simulink model "Punto4"  (R2025b)
settings: Solver=FixedStepAuto  StartTime=0.0  StopTime=60  FixedStep=1e-7  RelTol=1e-3
values from neighbouring files (symbols this model uses):
  A = zeros(2,2)    [Matlab_Traccia_B_(2).m]    (also in PROGETTO_CAT_TRACCIA_B_2.m; Punti_1_2_riscaldatore.m = [A11  A12; Punto_1_riscaldatore.m = [A11  A12; THEULTIMAEONE.m)
  B = zeros(2,1)    [Matlab_Traccia_B_(2).m]    (also in PROGETTO_CAT_TRACCIA_B_2.m; Punti_1_2_riscaldatore.m = [B1; Punto_1_riscaldatore.m = [B1; THEULTIMAEONE.m)
  C = [0 1]    [Matlab_Traccia_B_(2).m]    (also in PROGETTO_CAT_TRACCIA_B_2.m; Punti_1_2_riscaldatore.m; Punto_1_riscaldatore.m; THEULTIMAEONE.m)
  D = 0    [Matlab_Traccia_B_(2).m]    (also in PROGETTO_CAT_TRACCIA_B_2.m; Punti_1_2_riscaldatore.m; Punto_1_riscaldatore.m; THEULTIMAEONE.m)
libraries: cstblocks x1
settings Model: Creator=alex  LastModifiedBy=alex

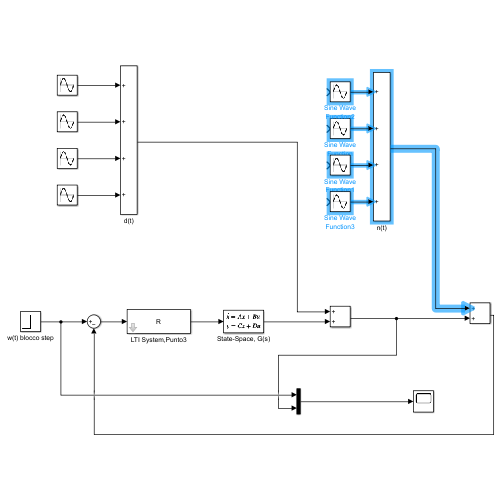
[thumbnail: Simulink's stored preview of the top-level diagram]
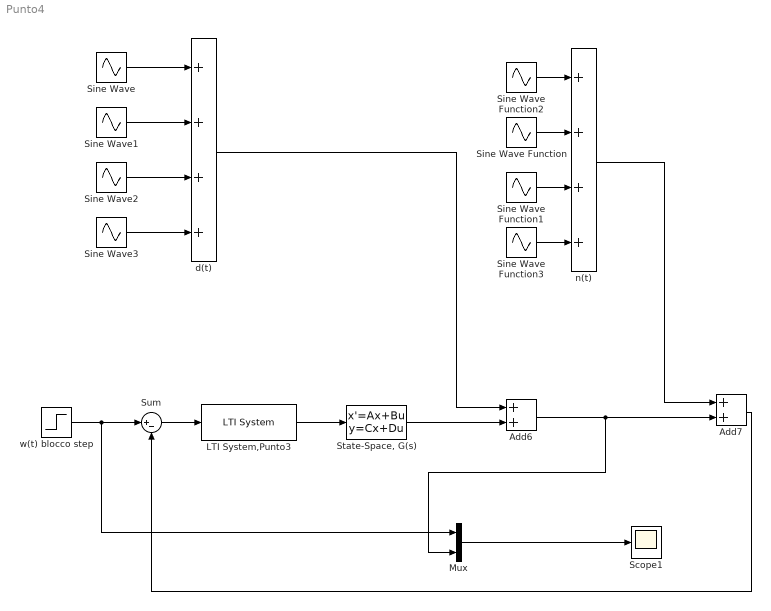
== system Punto4 ==
  Add6 : Sum
  Add7 : Sum
  LTI System,Punto3 : cstblocks/LTI System  sys=R  IC=[]  PadeOrder=0
  Mux : Mux  Inputs=2
  Scope1 : Scope
      settings: ActiveDisplayYMinimum=2.3064084257449133  ActiveDisplayYMaximum=3.4959386286082776  DataLoggingVariableName=sim_out
  Sine Wave : Sin  Amplitude=1.5  Frequency=0.08  SampleTime=0
  Sine Wave Function : Sin  TimeSource=Use external signal  Amplitude=0  Frequency=10e4  SampleTime=0
  Sine Wave Function1 : Sin  TimeSource=Use external signal  Amplitude=0  Frequency=15e4  SampleTime=0
  Sine Wave Function2 : Sin  TimeSource=Use external signal  Amplitude=0  Frequency=5e4  SampleTime=0
  Sine Wave Function3 : Sin  TimeSource=Use external signal  Amplitude=0  Frequency=20e4  SampleTime=0
  Sine Wave1 : Sin  Amplitude=1.5  Frequency=0.16  SampleTime=0
  Sine Wave2 : Sin  Amplitude=1.5  Frequency=0.24  SampleTime=0
  Sine Wave3 : Sin  Amplitude=1.5  Frequency=0.32  SampleTime=0
  "State-Space, G(s)" : StateSpace  A=A  B=B  C=C  D=D  InitialCondition=[0 0]
  Sum : Sum  Inputs=|+-
  d(t) : Sum  Inputs=++++
  n(t) : Sum  Inputs=++++
  w(t) blocco step : Step  Time=0  After=4  SampleTime=0
  wires:
  Sine Wave/1 -> d(t)/1
  Sine Wave1/1 -> d(t)/2
  Sine Wave3/1 -> d(t)/4
  Sine Wave Function2/1 -> n(t)/1
  Sine Wave Function/1 -> n(t)/2
  Sine Wave Function1/1 -> n(t)/3
  Sine Wave Function3/1 -> n(t)/4
  w(t) blocco step/1 -> Mux/1, Sum/1
  Sum/1 -> LTI System,Punto3/1
  LTI System,Punto3/1 -> "State-Space, G(s)"/1
  Add6/1 -> Add7/2, Mux/2
  Add7/1 -> Sum/2
  Mux/1 -> Scope1/1
  Sine Wave2/1 -> d(t)/3
  "State-Space, G(s)"/1 -> Add6/2
  d(t)/1 -> Add6/1
  n(t)/1 -> Add7/1
